simulink model "AircraftFeedbackControlLoop"  (R2023b)
settings: Solver=FixedStepDiscrete  StartTime=0.0  StopTime=12  FixedStep=Sample_time  RelTol=1e-3
undefined symbols (not defined in the file): actuator_filter_alpha, actuator_limit_deg, aircraft_control_effectiveness, aircraft_pitch_damping, controller_integrator_ic, DiscIntNeverNeededParam, initial_pitch_angle, initial_q_rate, pitch_Ki, pitch_Kp, Sample_time, sensor_filter_alpha
Description:
  | Illustrative 50 Hz closed-loop longitudinal training plant. The parameters are deliberately simplified and are not aircraft data.
settings Model: DataDictionary=FCS_Data.sldd  Creator=Tyler  LastModifiedBy=Tyler
settings CodeAppCC: MaxIdLength=63

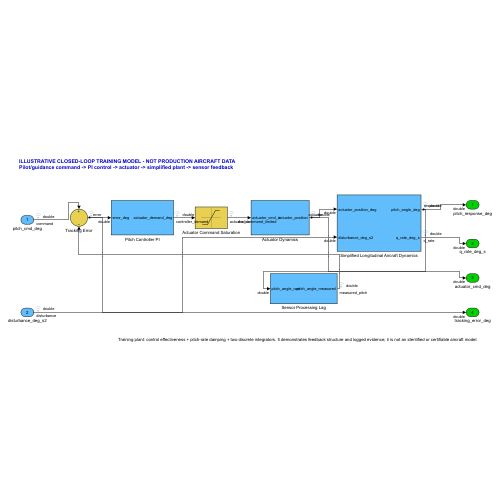
[thumbnail: Simulink's stored preview of the top-level diagram]
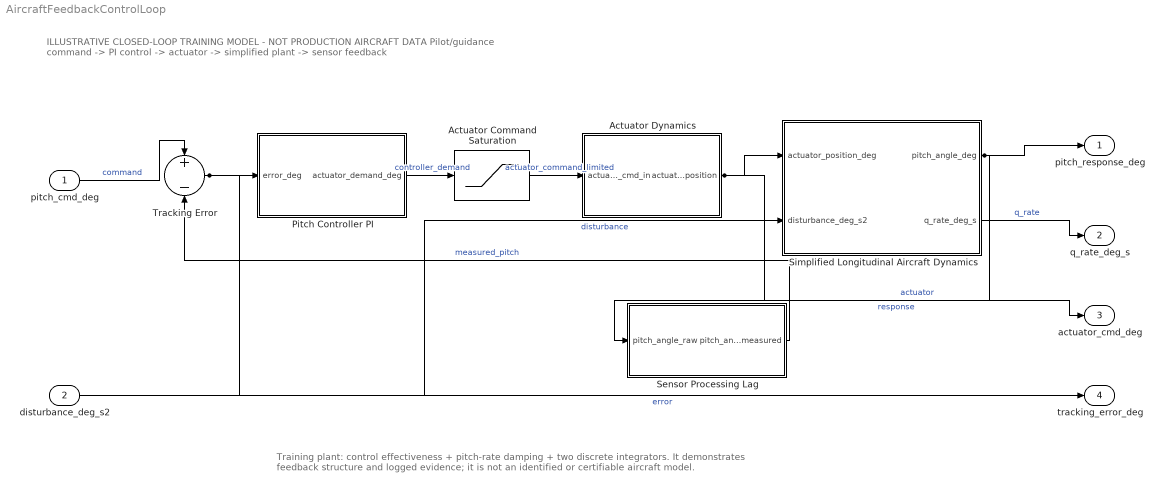
== system AircraftFeedbackControlLoop ==
  note: ILLUSTRATIVE CLOSED-LOOP TRAINING MODEL - NOT PRODUCTION AIRCRAFT DATA
      | Pilot/guidance command -> PI control -> actuator -> simplified plant -> sensor feedback
  note: Training plant: control effectiveness + pitch-rate damping + two discrete integrators. It demonstrates feedback structure and logged evidence; it is not an identified or certifiable aircraft model.
  pitch_cmd_deg : Inport  OutDataTypeStr=double  Unit=deg  SampleTime=Sample_time
  disturbance_deg_s2 : Inport  Port=2  OutDataTypeStr=double  Unit=deg/s^2  SampleTime=Sample_time
  Actuator Command Saturation : Saturate  UpperLimit=actuator_limit_deg  LowerLimit=-actuator_limit_deg
  Actuator Dynamics : Subsystem
  Pitch Controller PI : Subsystem
  Sensor Processing Lag : Subsystem
  Simplified Longitudinal Aircraft Dynamics : Subsystem
  Tracking Error : Sum  Inputs=+-
  pitch_response_deg : Outport  OutDataTypeStr=double  Unit=deg
  q_rate_deg_s : Outport  Port=2  OutDataTypeStr=double  Unit=deg/s
  actuator_cmd_deg : Outport  Port=3  OutDataTypeStr=double  Unit=deg
  tracking_error_deg : Outport  Port=4  OutDataTypeStr=double  Unit=deg
  wires:
  pitch_cmd_deg/1 -> Tracking Error/1  "command"
  Tracking Error/1 -> Pitch Controller PI/1(error_deg), tracking_error_deg/1  "error"
  Pitch Controller PI/1(actuator_demand_deg) -> Actuator Command Saturation/1  "controller_demand"
  Actuator Command Saturation/1 -> Actuator Dynamics/1(actuator_cmd_in)  "actuator_command_limited"
  Actuator Dynamics/1(actuator_position) -> Simplified Longitudinal Aircraft Dynamics/1(actuator_position_deg), actuator_cmd_deg/1  "actuator"
  disturbance_deg_s2/1 -> Simplified Longitudinal Aircraft Dynamics/2(disturbance_deg_s2)  "disturbance"
  Simplified Longitudinal Aircraft Dynamics/1(pitch_angle_deg) -> pitch_response_deg/1, Sensor Processing Lag/1(pitch_angle_raw)  "response"
  Sensor Processing Lag/1(pitch_angle_measured) -> Tracking Error/2  "measured_pitch"
  Simplified Longitudinal Aircraft Dynamics/2(q_rate_deg_s) -> q_rate_deg_s/1  "q_rate"

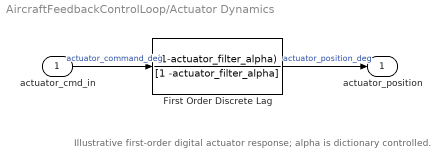
== system AircraftFeedbackControlLoop/Actuator Dynamics ==
  note: Illustrative first-order digital actuator response; alpha is dictionary controlled.
  actuator_cmd_in : Inport  OutDataTypeStr=double  Unit=deg  SampleTime=Sample_time
  First Order Discrete Lag : DiscreteTransferFcn  Numerator=(1-actuator_filter_alpha)  Denominator=[1 -actuator_filter_alpha]  SampleTime=Sample_time
  actuator_position : Outport  OutDataTypeStr=double  Unit=deg
  wires:
  actuator_cmd_in/1 -> First Order Discrete Lag/1  "actuator_command_deg"
  First Order Discrete Lag/1 -> actuator_position/1  "actuator_position_deg"

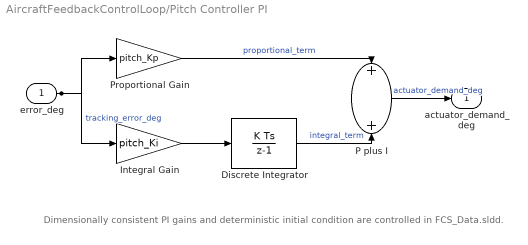
== system AircraftFeedbackControlLoop/Pitch Controller PI ==
  note: Dimensionally consistent PI gains and deterministic initial condition are controlled in FCS_Data.sldd.
  error_deg : Inport  OutDataTypeStr=double  Unit=deg  SampleTime=Sample_time
  Discrete Integrator : DiscreteIntegrator  gainval=1  InitialCondition=controller_integrator_ic  SampleTime=Sample_time  ICPrevOutput=DiscIntNeverNeededParam  ICPrevScaledInput=DiscIntNeverNeededParam
  Integral Gain : Gain  Gain=pitch_Ki
  P plus I : Sum
  Proportional Gain : Gain  Gain=pitch_Kp
  actuator_demand_deg : Outport  OutDataTypeStr=double  Unit=deg
  wires:
  error_deg/1 -> Proportional Gain/1, Integral Gain/1  "tracking_error_deg"
  Proportional Gain/1 -> P plus I/1  "proportional_term"
  Integral Gain/1 -> Discrete Integrator/1
  Discrete Integrator/1 -> P plus I/2  "integral_term"
  P plus I/1 -> actuator_demand_deg/1  "actuator_demand_deg"

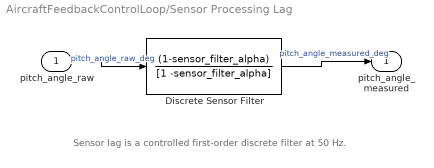
== system AircraftFeedbackControlLoop/Sensor Processing Lag ==
  note: Sensor lag is a controlled first-order discrete filter at 50 Hz.
  pitch_angle_raw : Inport  OutDataTypeStr=double  Unit=deg  SampleTime=Sample_time
  Discrete Sensor Filter : DiscreteTransferFcn  Numerator=(1-sensor_filter_alpha)  Denominator=[1 -sensor_filter_alpha]  SampleTime=Sample_time
  pitch_angle_measured : Outport  OutDataTypeStr=double  Unit=deg
  wires:
  pitch_angle_raw/1 -> Discrete Sensor Filter/1  "pitch_angle_raw_deg"
  Discrete Sensor Filter/1 -> pitch_angle_measured/1  "pitch_angle_measured_deg"

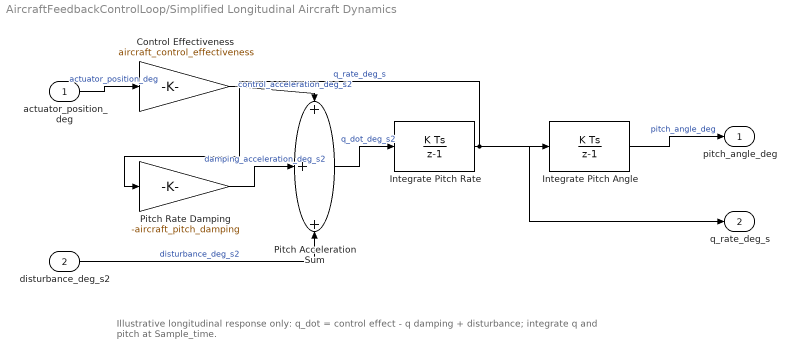
== system AircraftFeedbackControlLoop/Simplified Longitudinal Aircraft Dynamics ==
  note: Illustrative longitudinal response only: q_dot = control effect - q damping + disturbance; integrate q and pitch at Sample_time.
  actuator_position_deg : Inport  OutDataTypeStr=double  Unit=deg  SampleTime=Sample_time
  disturbance_deg_s2 : Inport  Port=2  OutDataTypeStr=double  Unit=deg/s^2  SampleTime=Sample_time
  Control Effectiveness : Gain  Gain=aircraft_control_effectiveness
  Integrate Pitch Angle : DiscreteIntegrator  gainval=1  InitialCondition=initial_pitch_angle  SampleTime=Sample_time  ICPrevOutput=DiscIntNeverNeededParam  ICPrevScaledInput=DiscIntNeverNeededParam
  Integrate Pitch Rate : DiscreteIntegrator  gainval=1  InitialCondition=initial_q_rate  SampleTime=Sample_time  ICPrevOutput=DiscIntNeverNeededParam  ICPrevScaledInput=DiscIntNeverNeededParam
  Pitch Acceleration Sum : Sum  Inputs=+++
  Pitch Rate Damping : Gain  Gain=-aircraft_pitch_damping
  pitch_angle_deg : Outport  OutDataTypeStr=double  Unit=deg
  q_rate_deg_s : Outport  Port=2  OutDataTypeStr=double  Unit=deg/s
  wires:
  actuator_position_deg/1 -> Control Effectiveness/1  "actuator_position_deg"
  Control Effectiveness/1 -> Pitch Acceleration Sum/1  "control_acceleration_deg_s2"
  Pitch Rate Damping/1 -> Pitch Acceleration Sum/2  "damping_acceleration_deg_s2"
  disturbance_deg_s2/1 -> Pitch Acceleration Sum/3  "disturbance_deg_s2"
  Pitch Acceleration Sum/1 -> Integrate Pitch Rate/1  "q_dot_deg_s2"
  Integrate Pitch Rate/1 -> Integrate Pitch Angle/1, Pitch Rate Damping/1, q_rate_deg_s/1  "q_rate_deg_s"
  Integrate Pitch Angle/1 -> pitch_angle_deg/1  "pitch_angle_deg"
